simulink model "RobotX_ss_acousticsSingle_DockT_1024"  (R2014a)
settings: Solver=FixedStepDiscrete  StartTime=0.0  StopTime=inf  FixedStep=.25  RelTol=1e-3
undefined symbols (not defined in the file): Com1, Com2, Com3, Com4, DiscIntNeverNeededParam, standard
libraries: xpcseriallib x42, slrtlib x7, simulink x6, speedgoatlib x2, dspmtrx3 x1, speedgoatlib_IO102 x1
(part 3 of 4)

== system RobotX_ss_acousticsSingle_DockT_1024/Sensors/1024 Comms/Pi Nav Send ==
  Parameters : Inport
  ASCII Encode 3 : xpcseriallib/ASCII Encode   format="{\"Valid\":%d, \"Mode\":%d, \"Length\":%d, \"Activate\":%d, \"Waypoints\":[%f, %f, %f, %f, %f, %f, %f, %f, %f, %f, %f, %f, %f, %f, %f, %f, %f, %f, %f, %f, %f, %f, %f, %f]} \\r\\n"  nvars=28  maxlength=1000  vartypes={ 'double' }
  Bus Selector : BusSelector  OutputSignals=Outputs.Navigation Outputs.Valid,Outputs.Navigation Outputs.Control Mode,Outputs.Navigation Outputs.Data,Outputs.Acoustic Active
  Data Update1 : MATLAB Function  Commented=on  TreatAsAtomicUnit=on
  Data Update2 : MATLAB Function  TreatAsAtomicUnit=on
  LCM Complete Encode : xpcseriallib/ASCII Encode   Commented=on  format="{\"Valid\":%d, \"Mode\":%d, \"Length\":%d, \"Activate\":%d, \"Waypoints\":[%f, %f, %f, %f, %f, %f, %f, %f, %f, %f, %f, %f, %f, %f, %f, %f, %f, %f, %f, %f, %f, %f, %f, %f]} \\r\\n"  nvars=28  maxlength=1000  vartypes={ 'double' }
  Serial Send : Outport
  wires:
  Parameters/1 -> Bus Selector/1
  ASCII Encode 3/1 -> Serial Send/1
  Bus Selector/1 -> Data Update2/1(Valid)  "<Valid>"
  Bus Selector/2 -> Data Update2/2(ControlMode)  "<Control Mode>"
  Bus Selector/3 -> Data Update2/3(Data)  "<Data>"
  Data Update2/21(D17) -> ASCII Encode 3/21
  Data Update2/20(D16) -> ASCII Encode 3/20
  Data Update2/19(D15) -> ASCII Encode 3/19
  Data Update2/4(A) -> ASCII Encode 3/4
  Data Update2/2(C) -> ASCII Encode 3/2
  Data Update2/18(D14) -> ASCII Encode 3/18
  Data Update2/16(D12) -> ASCII Encode 3/16
  Data Update2/7(D3) -> ASCII Encode 3/7
  Data Update2/6(D2) -> ASCII Encode 3/6
  Data Update2/5(D1) -> ASCII Encode 3/5
  Data Update2/17(D13) -> ASCII Encode 3/17
  Data Update2/9(D5) -> ASCII Encode 3/9
  Data Update2/10(D6) -> ASCII Encode 3/10
  Data Update2/24(D20) -> ASCII Encode 3/24
  Data Update2/23(D19) -> ASCII Encode 3/23
  Data Update2/28(D24) -> ASCII Encode 3/28
  Data Update2/26(D22) -> ASCII Encode 3/26
  Data Update2/25(D21) -> ASCII Encode 3/25
  Data Update2/3(L) -> ASCII Encode 3/3
  Data Update2/27(D23) -> ASCII Encode 3/27
  Data Update2/8(D4) -> ASCII Encode 3/8
  Data Update2/11(D7) -> ASCII Encode 3/11
  Data Update2/13(D9) -> ASCII Encode 3/13
  Data Update2/12(D8) -> ASCII Encode 3/12
  Data Update2/14(D10) -> ASCII Encode 3/14
  Data Update2/22(D18) -> ASCII Encode 3/22
  Data Update2/15(D11) -> ASCII Encode 3/15
  Bus Selector/4 -> Data Update2/4(Activate)  "<Acoustic Active>"
  Data Update2/1(V) -> ASCII Encode 3/1
  Data Update1/1(V) -> LCM Complete Encode/1
  Data Update1/2(C) -> LCM Complete Encode/2
  Data Update1/6(D2) -> LCM Complete Encode/6
  Data Update1/7(D3) -> LCM Complete Encode/7
  Data Update1/8(D4) -> LCM Complete Encode/8
  Data Update1/5(D1) -> LCM Complete Encode/5
  Data Update1/9(D5) -> LCM Complete Encode/9
  Data Update1/10(D6) -> LCM Complete Encode/10
  Data Update1/11(D7) -> LCM Complete Encode/11
  Data Update1/12(D8) -> LCM Complete Encode/12
  Data Update1/13(D9) -> LCM Complete Encode/13
  Data Update1/18(D14) -> LCM Complete Encode/18
  Data Update1/15(D11) -> LCM Complete Encode/15
  Data Update1/20(D16) -> LCM Complete Encode/20
  Data Update1/21(D17) -> LCM Complete Encode/21
  Data Update1/19(D15) -> LCM Complete Encode/19
  Data Update1/14(D10) -> LCM Complete Encode/14
  Data Update1/16(D12) -> LCM Complete Encode/16
  Data Update1/22(D18) -> LCM Complete Encode/22
  Data Update1/23(D19) -> LCM Complete Encode/23
  Data Update1/24(D20) -> LCM Complete Encode/24
  Data Update1/25(D21) -> LCM Complete Encode/25
  Data Update1/27(D23) -> LCM Complete Encode/27
  Data Update1/26(D22) -> LCM Complete Encode/26
  Data Update1/28(D24) -> LCM Complete Encode/28
  Data Update1/3(L) -> LCM Complete Encode/3
  Data Update1/4(A) -> LCM Complete Encode/4
  Data Update1/17(D13) -> LCM Complete Encode/17

== system RobotX_ss_acousticsSingle_DockT_1024/Sensors/1024 Comms/Subsystem ==
  Bus Creator : BusCreator  Inputs=3
  Bus Creator1 : BusCreator  Inputs=2
  Bus Creator2 : BusCreator  Inputs=2
  Constant : Constant  Value=zeros(12,1)
  Constant1 : Constant  Value=zeros(12,1)
  Constant2 : Constant  Value=zeros(4,1)
  Constant3 : Constant  Value=zeros(4,1)
  Constant4 : Constant  Value=zeros(4,1)
  Fake Panda : Outport
  wires:
  Constant/1 -> Bus Creator1/1  "Distances"
  Constant1/1 -> Bus Creator1/2  "Angles"
  Constant2/1 -> Bus Creator/1  "Color"
  Constant3/1 -> Bus Creator/2  "Probability"
  Constant4/1 -> Bus Creator/3  "idx"
  Bus Creator1/1 -> Bus Creator2/1  "Landmarks"
  Bus Creator/1 -> Bus Creator2/2  "Color data"
  Bus Creator2/1 -> Fake Panda/1  "Lidar Data Input"

== system RobotX_ss_acousticsSingle_DockT_1024/Sensors/1024 Comms/UTC Timer ==
  Start Time : Inport
  MATLAB Function : MATLAB Function  TreatAsAtomicUnit=on
  Real Time : Outport
  wires:
  Start Time/1 -> MATLAB Function/1(inTime)
  MATLAB Function/1(timeOut) -> Real Time/1

== system RobotX_ss_acousticsSingle_DockT_1024/Sensors/1024 Comms/data log ==
  Sensors signal : Inport
  Bus to Vector : BusToVector
  Read : DataStoreRead  DataStoreName=PingPose
  Scope 2 : slrtlib/Displays and Logging/Scope   scopeno=2  scopetype=File  autostart=on  viewmode=Graphical redraw  formatstr='%15.6f'  grid=on  ylimits=[0,0]  nosamples=250  noprepostsamples=0  interleave=1  triggermode=FreeRun  triggersignal=1  trigsignalfromport=off  triggerlevel=0.0  triggerslope=Either  triggerscope=1  triggersample=0  filename=NAL1_<%%%>1.dat  mode=Commit  writesize=512  autorestart=on  dynamicfilemode=on  maxwritefilesize=512*1024^2
  Scope 4 : slrtlib/Displays and Logging/Scope   scopeno=1  scopetype=File  autostart=on  viewmode=Graphical redraw  formatstr='%15.6f'  grid=on  ylimits=[0,0]  nosamples=250  noprepostsamples=0  interleave=1  triggermode=FreeRun  triggersignal=1  trigsignalfromport=off  triggerlevel=0.0  triggerslope=Either  triggerscope=1  triggersample=0  filename=pPos_<%%%>1.dat  mode=Commit  writesize=512  autorestart=on  dynamicfilemode=on  maxwritefilesize=512*1024^2
  wires:
  Sensors signal/1 -> Bus to Vector/1
  Bus to Vector/1 -> Scope 2/1
  Read/1 -> Scope 4/1

== system RobotX_ss_acousticsSingle_DockT_1024/Main FSM/Acoustic Single Point FSM/Acoustics Orient/Output Heirarchy ==
  Data : Inport
  Sensors : Inport  Port=2
  Acoustic Active : Constant
  Bus Creator2 : BusCreator  Inputs=3
  Bus Creator3 : BusCreator  Inputs=3
  Bus Creator5 : BusCreator  Inputs=2
  Constant : Constant
  Constant3 : Constant
  Lidar Mode : Constant
  Outputs : Outport
  wires:
  Sensors/1 -> Bus Creator5/2  "Sensors"
  Bus Creator5/1 -> Outputs/1  "Output Signals"
  Constant/1 -> Bus Creator2/1  "Valid"
  Constant3/1 -> Bus Creator2/2  "Control Mode"
  Data/1 -> Bus Creator2/3  "Data"
  Bus Creator2/1 -> Bus Creator3/1  "Navigation Outputs"
  Acoustic Active/1 -> Bus Creator3/2  "Acoustic Active"
  Lidar Mode/1 -> Bus Creator3/3  "Lidar Mode"
  Bus Creator3/1 -> Bus Creator5/1  "Outputs"

== system RobotX_ss_acousticsSingle_DockT_1024/Main FSM/Acoustic Single Point FSM/Move/Output Reassign ==
  Vaild : Inport
  Data : Inport  Port=2
  Sensors : Inport  Port=3
  Acoustic Active : Constant  Value=0
  Bus Creator2 : BusCreator  Inputs=3
  Bus Creator3 : BusCreator  Inputs=3
  Bus Creator5 : BusCreator  Inputs=2
  Constant3 : Constant  Value=0
  Lidar Mode : Constant  Value=0
  Outputs : Outport
  wires:
  Sensors/1 -> Bus Creator5/2  "Sensors"
  Bus Creator5/1 -> Outputs/1  "Output Signals"
  Vaild/1 -> Bus Creator2/1  "Valid"
  Constant3/1 -> Bus Creator2/2  "Control Mode"
  Data/1 -> Bus Creator2/3  "Data"
  Bus Creator2/1 -> Bus Creator3/1  "Navigation Outputs"
  Acoustic Active/1 -> Bus Creator3/2  "Acoustic Active"
  Lidar Mode/1 -> Bus Creator3/3  "Lidar Mode"
  Bus Creator3/1 -> Bus Creator5/1  "Outputs"

== system RobotX_ss_acousticsSingle_DockT_1024/Main FSM/Acoustic Single Point FSM/Report/Output Heirarchy ==
  Sensors : Inport
  Data : Inport  Port=2
  Acoustic Active : Constant
  Bus Creator2 : BusCreator  Inputs=3
  Bus Creator3 : BusCreator  Inputs=3
  Bus Creator5 : BusCreator  Inputs=2
  Constant : Constant
  Constant3 : Constant
  Lidar Mode : Constant
  Outputs : Outport
  wires:
  Sensors/1 -> Bus Creator5/2  "Sensors"
  Bus Creator5/1 -> Outputs/1  "Output Signals"
  Constant/1 -> Bus Creator2/1  "Valid"
  Constant3/1 -> Bus Creator2/2  "Control Mode"
  Data/1 -> Bus Creator2/3  "Data"
  Bus Creator2/1 -> Bus Creator3/1  "Navigation Outputs"
  Acoustic Active/1 -> Bus Creator3/2  "Acoustic Active"
  Lidar Mode/1 -> Bus Creator3/3  "Lidar Mode"
  Bus Creator3/1 -> Bus Creator5/1  "Outputs"

== system RobotX_ss_acousticsSingle_DockT_1024/Main FSM/Docking/Docking/Output Heirarchy ==
  Data : Inport
  Sensors : Inport  Port=2
  Acoustic Active : Constant  Value=0
  Bus Creator2 : BusCreator  Inputs=3
  Bus Creator3 : BusCreator  Inputs=3
  Bus Creator5 : BusCreator  Inputs=2
  Constant : Constant
  Constant3 : Constant
  Lidar Mode : Constant  Value=2
  Outputs : Outport
  wires:
  Sensors/1 -> Bus Creator5/2  "Sensors"
  Bus Creator5/1 -> Outputs/1  "Output Signals"
  Constant/1 -> Bus Creator2/1  "Valid"
  Constant3/1 -> Bus Creator2/2  "Control Mode"
  Data/1 -> Bus Creator2/3  "Data"
  Bus Creator2/1 -> Bus Creator3/1  "Navigation Outputs"
  Acoustic Active/1 -> Bus Creator3/2  "Acoustic Active"
  Lidar Mode/1 -> Bus Creator3/3  "Lidar Mode"
  Bus Creator3/1 -> Bus Creator5/1  "Outputs"

== system RobotX_ss_acousticsSingle_DockT_1024/Main FSM/Docking/GPS Move/Output Reassign ==
  Vaild : Inport
  Data : Inport  Port=2
  Sensors : Inport  Port=3
  Acoustic Active : Constant  Value=0
  Bus Creator2 : BusCreator  Inputs=3
  Bus Creator3 : BusCreator  Inputs=3
  Bus Creator5 : BusCreator  Inputs=2
  Constant3 : Constant  Value=0
  Lidar Mode : Constant  Value=0
  Outputs : Outport
  wires:
  Sensors/1 -> Bus Creator5/2  "Sensors"
  Bus Creator5/1 -> Outputs/1  "Output Signals"
  Vaild/1 -> Bus Creator2/1  "Valid"
  Constant3/1 -> Bus Creator2/2  "Control Mode"
  Data/1 -> Bus Creator2/3  "Data"
  Bus Creator2/1 -> Bus Creator3/1  "Navigation Outputs"
  Acoustic Active/1 -> Bus Creator3/2  "Acoustic Active"
  Lidar Mode/1 -> Bus Creator3/3  "Lidar Mode"
  Bus Creator3/1 -> Bus Creator5/1  "Outputs"

== system RobotX_ss_acousticsSingle_DockT_1024/Main FSM/Docking/Reverse/Output Heirarchy ==
  Sensors : Inport
  Acoustic Active : Constant  Value=0
  Bus Creator2 : BusCreator  Inputs=3
  Bus Creator3 : BusCreator  Inputs=3
  Bus Creator5 : BusCreator  Inputs=2
  Constant2 : Constant  Value=[-100; -100; zeros(22,1)]
  Constant3 : Constant
  Constant4 : Constant  Value=2
  Lidar Mode : Constant  Value=2
  Outputs : Outport
  wires:
  Sensors/1 -> Bus Creator5/2  "Sensors"
  Bus Creator5/1 -> Outputs/1  "Output Signals"
  Constant3/1 -> Bus Creator2/1  "Valid"
  Constant4/1 -> Bus Creator2/2  "Control Mode"
  Constant2/1 -> Bus Creator2/3  "Data"
  Bus Creator2/1 -> Bus Creator3/1  "Navigation Outputs"
  Acoustic Active/1 -> Bus Creator3/2  "Acoustic Active"
  Lidar Mode/1 -> Bus Creator3/3  "Lidar Mode"
  Bus Creator3/1 -> Bus Creator5/1  "Outputs"

== matlab function RobotX_ss_acousticsSingle_DockT_1024/Main FSM/Docking/Docking/MATLAB Function ==
  data: QuayHeading input; TargetPoints input; Finished output; X input; Data output; Y input; Psi input; Dist input; Angles input; Prob input; Time input; dockNum input
function [Finished,Data] = Orient(QuayHeading,TargetPoints,X,Y,Psi,Dist,Angles,Prob,Time,dockNum)
%Written by Dylan DeGaetano on September 2, 2014
%Last Edited By Anderson Lebbad on September 19 2014

%This function passes the current pose data with the requrested heading
%so that the boat is facing the Quay wall.This task must be in station
%keeping mode
%
%Anderson's edit moved the orient within this function and adjusts the code
%to work better with sensing information

% 10/21 Edit: Correlates the estimated NED coord of the found symbol with
% known locations found through Ivan's map and proceeds to those locations

% Input TargetPoint is a 10x2 matrix of NED coords structured as follows
% [Observation Point; Dock1Start; Dock1Inter; Dock1Fin; Dock2Start;
% Dock2Inter; Dock2Fin; Dock3Start; Dock3Inter; Dock3Fin] where the bay
% numbers go from left to right

%work aound for communication issue
idx = Prob(4);
% Holdpose = station keeping point that we want to get to
% Pose = which waypoint to head to
% posIdx = which docking symbol position it is @
% 1 = Left, 2 = Middle, 3 = Right
% recognized = flag for if position of dock is found

persistent holdPose pos posIdx recognized

% If not to hold position
if isempty(holdPose)
    holdPose = [TargetPoints(1,:) QuayHeading]; % Initialize with Observation Points
    pos = 0;
    posIdx = 0;
    recognized = 0;
end

DistM=Dist(1)/100; % CM to M
Finished = 0; % Task not completed

%Initialize Data variable
Data = zeros(24,1); % 24x1 Array of Zeros


if idx(1) ~= 0 && recognized == 0
    %Calculate the NED coordinate of the found symbol
    TargetX = X+DistM(idx(1))*cos((Psi+Angles(idx(1)))*pi/180);
    TargetY = Y+DistM(idx(1))*sin((Psi+Angles(idx(1)))*pi/180);
    
    % Since the quay wall is very well aligned with EW directions,
    % correlate the estimated E coord of the found symbol with one of
    % the known bay positions
    bayEPos = [TargetPoints(4,2); TargetPoints(7,2); TargetPoints(10,2)];
    PosDiff = bayEPos - TargetY;
    [~,posIdx] = min(PosDiff);
    
    % Flag symbol as recognized
    recognized = 1; % Ensure that this calculation is not made again after the dock symbol pos is found/calculated
    
    % Begin proceeding to first position
    pos = 1;
end

if pos == 1
        %Set destination in front of dock to line up
        holdPose(1) = TargetPoints(pos+posIdx+2^(posIdx-1),1); % North
        holdPose(2) = TargetPoints(pos+posIdx+2^(posIdx-1),2); % East
    
    l1norm = abs(X-holdPose(1))+abs(Y-holdPose(2)); % calculate range to point we want to get to
    
    if l1norm < 2 % 2 metters
        % If within range, then flag first position complete and begin
        % proceeding to the hext position
        pos = 2;
    end
elseif pos == 2
        % Set intermediate point between start and finish
        holdPose(1) = TargetPoints(pos+posIdx+2^(posIdx-1),1); % North
        holdPose(2) = TargetPoints(pos+posIdx+2^(posIdx-1),2); % East
    
    l2norm = abs(X-holdPose(1)) + abs(Y-holdPose(2));
    
    if l2norm < 2
        % If within range, then flag second position complete and begin
        % proceeding to the hext position
        pos = 3;
    end
elseif pos == 3
        % Set final docking point
        holdPose(1) = TargetPoints(pos+posIdx+2^(posIdx-1),1); % North
        holdPose(2) = TargetPoints(pos+posIdx+2^(posIdx-1),2); % East
    
    l3norm = abs(X-holdPose(1)) + abs(Y-holdPose(2));
    
    if l3norm < 2
        holdPose = [X Y QuayHeading];
        Finished = 1;
    end
end

if Time >= 120 && recognized == 0
    % If symbol cannot be found within 60 seconds, proceed to middle bay
    posIdx = dockNum;
    recognized = 1;
end

holdPose(3) = QuayHeading;

Data(1) = holdPose(1);
Data(2) = holdPose(2);
Data(3) = holdPose(3);

== matlab function RobotX_ss_acousticsSingle_DockT_1024/Sensors/1020 Comms/MATLAB Function1 ==
  data: Valid input; Time input; asciiSEA output; Lat input; Long input; Color input; Depth input
% This function creates the underwater search message to be sent from 
% Speedgoat in ascii code
% Written by: Edward Zhu
% Date: 9/17/14

function asciiSEA = asciiSEAEncoder(Valid, Time, Lat, Long, Color, Depth)

% Initialize output message vector as the serial output block expects 128
% character message
asciiSEA = uint8(zeros(1,128));

% Convert static strings to ascii code
asciiMsgID = uint8('$RXSEA,');
asciiComma = uint8(',');
asciiDeciPt = uint8('.');
if Valid == 1
    if Lat >= 0
        asciiNS = uint8('N,');
    else
        Lat = -Lat;
        asciiNS = uint8('S,');
    end
    if Long >= 0
        asciiEW = uint8('E,');
    else
        Long = -Long;
        asciiEW = uint8('W,');
    end
else
    asciiNS = [32 asciiComma];
    asciiEW = [32 asciiComma];
end
asciiTeamID = uint8('FAUVU,');
asciiMsgEnd = uint8('*');
asciiMsgCRLF = [13 10];

% Convert UTC Time input (hhmmss) into ascii code
asciiTime = uint8(zeros(1,7));
asciiTime(7) = asciiComma;

for timeChar = 1:6
    asciiTime(timeChar) = floor(mod(Time,10^(7-timeChar))/...
        10^(6-timeChar)) + 48;
end

% Convert buoy color to ascii code (1 = R, 2 = G, 3 = B, 4 = W, 5 = K)
asciiColor = [uint8(32) asciiComma]; % Initialize as whitespace in case no buoy is found
if Valid == 1
    if Color == 1
        asciiColor(1) = uint8('R');
    elseif Color == 2
        asciiColor(1) = uint8('G');
    elseif Color == 3
        asciiColor(1) = uint8('B');
    elseif Color == 4
        asciiColor(1) = uint8('W');
    elseif Color == 5
        asciiColor(1) = uint8('K');
    end
end
% Convert latitude (dd.mmmmmm) into ascii code
asciiLat = uint8(zeros(1,10)+32); % Initialize as whitespace in case no buoy is found
asciiLat(10) = asciiComma;

% Only output values if valid bit is high
if Valid == 1
    asciiLat(3) = asciiDeciPt;
    latInt = floor(Lat);
    for latIntChar = 1:2
        asciiLat(latIntChar) = floor(mod(latInt,10^(3-latIntChar))/...
            10^(2-latIntChar)) + 48;
    end
    
    latDeci = mod(Lat,latInt) * 10^6;
    for latDeciChar = 1:6
        asciiLat(latDeciChar+3) = floor(mod(latDeci,10^(7-latDeciChar))/...
            10^(6-latDeciChar)) + 48;
    end
end

% Convert longitude (ddd.mmmmmm) into ascii code
asciiLong = uint8(zeros(1,11)+32); % Initialize as whitespace in case no buoy is found
asciiLong(11) = asciiComma;

% Only output values if valid bit is high
if Valid == 1
    asciiLong(4) = asciiDeciPt;
    longInt = floor(Long);
    for longIntChar = 1:3
        asciiLong(longIntChar) = floor(mod(longInt,10^(4-longIntChar))/...
            10^(3-longIntChar)) + 48;
    end
    
    longDeci = mod(Long,longInt) * 10^6;
    for longDeciChar = 1:6
        asciiLong(longDeciChar+4) = floor(mod(longDeci,10^(7-longDeciChar))/...
            10^(6-longDeciChar)) + 48;
    end
end

% Convert depth (m) (##.##) into ascii
asciiDepth = uint8(zeros(1,6)+32); % Initialize as whitespace in case no buoy is found
asciiDepth(6) = asciiMsgEnd;

% Only output values if valid bit is high
if Valid == 1
    asciiDepth(3) = asciiDeciPt;
    depthInt = floor(Depth);
    for depthIntChar = 1:2
        asciiDepth(depthIntChar) = floor(mod(depthInt,10^(3-depthIntChar))/...
            10^(2-depthIntChar)) + 48;
    end
    
    depthDeci = mod(Depth,depthInt) * 10^2;
    for depthDeciChar = 1:2
        asciiDepth(depthDeciChar+3) = floor(mod(depthDeci,10^(3-depthDeciChar))/...
            10^(2-depthDeciChar)) + 48;
    end
end

% Concat individual ascii arrays into one array
asciiPreChkSum = cat(2,asciiMsgID,asciiTime,asciiTeamID,asciiColor,...
    asciiLat,asciiNS,asciiLong,asciiEW,asciiDepth);

% Calculate the checksum of the message from the '$' to the '*' and convert
% to hex
chkSum = uint8(0);

for chksumChar = 1:(length(asciiPreChkSum)-2)
    chkSum = bitxor(chkSum,asciiPreChkSum(chksumChar+1));
end

% Convert the checksum to ascii
chkSum = dec2hex(chkSum);
asciiChkSum = uint8(zeros(1,length(chkSum))+32);
for i = 1:length(chkSum)
    asciiChkSum(i) = uint8(chkSum(i));
end

% Concat the checksum and the '/r/n' to the end of the message
asciiPostChkSum = cat(2,asciiPreChkSum,asciiChkSum,asciiMsgCRLF);

% Output the final message
asciiSEA(1:length(asciiPostChkSum)) = asciiPostChkSum;

== system RobotX_ss_acousticsSingle_DockT_1024/Main FSM/Start//Speedgate/Aim/Output Heirarchy ==
  Data : Inport
  Sensors : Inport  Port=2
  Acoustic Active : Constant  Value=0
  Bus Creator2 : BusCreator  Inputs=3
  Bus Creator3 : BusCreator  Inputs=3
  Bus Creator5 : BusCreator  Inputs=2
  Constant : Constant
  Constant3 : Constant
  Lidar Mode : Constant
  Outputs : Outport
  wires:
  Sensors/1 -> Bus Creator5/2  "Sensors"
  Bus Creator5/1 -> Outputs/1  "Output Signals"
  Constant/1 -> Bus Creator2/1  "Valid"
  Constant3/1 -> Bus Creator2/2  "Control Mode"
  Data/1 -> Bus Creator2/3  "Data"
  Bus Creator2/1 -> Bus Creator3/1  "Navigation Outputs"
  Acoustic Active/1 -> Bus Creator3/2  "Acoustic Active"
  Lidar Mode/1 -> Bus Creator3/3  "Lidar Mode"
  Bus Creator3/1 -> Bus Creator5/1  "Outputs"

== system RobotX_ss_acousticsSingle_DockT_1024/Main FSM/Start//Speedgate/Dead Reckon/Output Reassign ==
  Vaild : Inport
  Data : Inport  Port=2
  Sensors : Inport  Port=3
  Acoustic Active : Constant  Value=0
  Bus Creator2 : BusCreator  Inputs=3
  Bus Creator3 : BusCreator  Inputs=3
  Bus Creator5 : BusCreator  Inputs=2
  Constant3 : Constant  Value=0
  Lidar Mode : Constant  Value=3
  Outputs : Outport
  wires:
  Sensors/1 -> Bus Creator5/2  "Sensors"
  Bus Creator5/1 -> Outputs/1  "Output Signals"
  Vaild/1 -> Bus Creator2/1  "Valid"
  Constant3/1 -> Bus Creator2/2  "Control Mode"
  Data/1 -> Bus Creator2/3  "Data"
  Bus Creator2/1 -> Bus Creator3/1  "Navigation Outputs"
  Acoustic Active/1 -> Bus Creator3/2  "Acoustic Active"
  Lidar Mode/1 -> Bus Creator3/3  "Lidar Mode"
  Bus Creator3/1 -> Bus Creator5/1  "Outputs"

== system RobotX_ss_acousticsSingle_DockT_1024/Main FSM/Start//Speedgate/GPS Move/Output Reassign ==
  Vaild : Inport
  Data : Inport  Port=2
  Sensors : Inport  Port=3
  Acoustic Active : Constant  Value=0
  Bus Creator2 : BusCreator  Inputs=3
  Bus Creator3 : BusCreator  Inputs=3
  Bus Creator5 : BusCreator  Inputs=2
  Constant3 : Constant  Value=0
  Lidar Mode : Constant  Value=0
  Outputs : Outport
  wires:
  Sensors/1 -> Bus Creator5/2  "Sensors"
  Bus Creator5/1 -> Outputs/1  "Output Signals"
  Vaild/1 -> Bus Creator2/1  "Valid"
  Constant3/1 -> Bus Creator2/2  "Control Mode"
  Data/1 -> Bus Creator2/3  "Data"
  Bus Creator2/1 -> Bus Creator3/1  "Navigation Outputs"
  Acoustic Active/1 -> Bus Creator3/2  "Acoustic Active"
  Lidar Mode/1 -> Bus Creator3/3  "Lidar Mode"
  Bus Creator3/1 -> Bus Creator5/1  "Outputs"

== system RobotX_ss_acousticsSingle_DockT_1024/Sensors/1024 Comms/Message Selector/HRT Message ==
  Parameters : Inport
  Time : Inport  Port=2
  Bus Selector : BusSelector  OutputSignals=Sensors.Navigation Message.GPS (LLA).Lat,Sensors.Navigation Message.GPS (LLA).Long,Sensors.Navigation Message.On/Off/RC/Auto,Main Task
  MATLAB Function : MATLAB Function  TreatAsAtomicUnit=on
  HRT Message : Outport
  wires:
  MATLAB Function/1(asciiHRT) -> HRT Message/1
  Parameters/1 -> Bus Selector/1
  Time/1 -> MATLAB Function/1(Time)
  Bus Selector/1 -> MATLAB Function/2(HRTLat)  "<Lat>"
  Bus Selector/2 -> MATLAB Function/3(HRTLong)  "<Long>"
  Bus Selector/3 -> MATLAB Function/4(HRTMode)  "<On/Off/RC/Auto>"
  Bus Selector/4 -> MATLAB Function/5(HRTTask)  "<Main Task>"

== system RobotX_ss_acousticsSingle_DockT_1024/Sensors/1024 Comms/Message Selector/HRTLIT Message ==
  Parameters : Inport
  Time : Inport  Port=2
  Bus Selector : BusSelector  OutputSignals=Sensors.Navigation Message.GPS (LLA).Lat,Sensors.Navigation Message.GPS (LLA).Long,Main Task,Sensors.Navigation Message.On/Off/RC/Auto
  Data Store Read1 : DataStoreRead  DataStoreName=ltSeq
  MATLAB Function : MATLAB Function  TreatAsAtomicUnit=on
  MATLAB Function1 : MATLAB Function  TreatAsAtomicUnit=on
  HRTLIT Message : Outport
  wires:
  MATLAB Function/1(asciiHRTLIT) -> HRTLIT Message/1
  Time/1 -> MATLAB Function/1(Time)
  Parameters/1 -> Bus Selector/1
  Bus Selector/3 -> MATLAB Function/4(HRTTask)  "<Main Task>"
  Bus Selector/2 -> MATLAB Function/3(HRTLong)  "<Long>"
  Bus Selector/1 -> MATLAB Function/2(HRTLat)  "<Lat>"
  Bus Selector/4 -> MATLAB Function/5(HRTMode)  "<On/Off/RC/Auto>"
  Data Store Read1/1 -> MATLAB Function1/1(ltSeq)
  MATLAB Function1/2(LITSequence) -> MATLAB Function/7(LITSequence)
  MATLAB Function1/1(LITValid) -> MATLAB Function/6(LITValid)

== system RobotX_ss_acousticsSingle_DockT_1024/Sensors/1024 Comms/Message Selector/HRTSEA Message ==
  Parameters : Inport
  Time : Inport  Port=2
  Bus Selector : BusSelector  OutputSignals=Sensors.Navigation Message.GPS (LLA).Lat,Sensors.Navigation Message.GPS (LLA).Long,Main Task,Sensors.Navigation Message.On/Off/RC/Auto
  Data Store Read3 : DataStoreRead  DataStoreName=pingerInfo
  MATLAB Function : MATLAB Function  TreatAsAtomicUnit=on
  MATLAB Function1 : MATLAB Function  TreatAsAtomicUnit=on
  HRTSEA Message : Outport
  wires:
  MATLAB Function/1(asciiHRTSEA) -> HRTSEA Message/1
  Parameters/1 -> Bus Selector/1
  Time/1 -> MATLAB Function/1(Time)
  Data Store Read3/1 -> MATLAB Function1/1(pingerInfo)
  Bus Selector/3 -> MATLAB Function/4(HRTTask)  "<Main Task>"
  Bus Selector/1 -> MATLAB Function/2(HRTLat)  "<Lat>"
  Bus Selector/2 -> MATLAB Function/3(HRTLong)  "<Long>"
  Bus Selector/4 -> MATLAB Function/5(HRTMode)  "<On/Off/RC/Auto>"
  MATLAB Function1/3(SEALong) -> MATLAB Function/8(SEALong)
  MATLAB Function1/2(SEALat) -> MATLAB Function/7(SEALat)
  MATLAB Function1/5(SEADepth) -> MATLAB Function/10(SEADepth)
  MATLAB Function1/4(SEAColor) -> MATLAB Function/9(SEAColor)
  MATLAB Function1/1(SEAValid) -> MATLAB Function/6(SEAValid)

== matlab function RobotX_ss_acousticsSingle_DockT_1024/Main FSM/Acoustic Single Point FSM/Report/writePingInfo ==
  data: acouX input; acouY input; Depth input; NED_Origin input; pingerInfo output; AcousticPose1 input; colorQuad input
function pingerInfo = writePingInfo(acouX,acouY,Depth,NED_Origin,AcousticPose1,colorQuad)
%Written By Anderson Lebbad on October 22, 2014
%Last Edited By:
%
%This function takes the info from the acoustic pose to create an estimate
%of pinger position in North East Down coordinates, then converts that to
%LLA. From here, a buoy color is chosen based off the quadrant, and the
%info is formatted for the message writing block - including the valid bit.

Psi = AcousticPose1(3);

%Quadrants -
%NE : 1
%SE : 2
%SW : 3
%NW : 4
Quad = round((mod(Psi,360)+45)/90);



%Color code-
%R : 1
%G : 2
%B : 3
%W : 4
%K : 5

switch Quad
    case 1
        color = colorQuad(1);
    case 2
        color = colorQuad(2);
    case 3
        color = colorQuad(3);
    otherwise
        color = colorQuad(4);
end

%Convert to LLA
LLA = ecef2lla(ned2ecef(NED_Origin'*pi/180,[acouX; acouY; 0]))*180/pi;

%Output
pingerInfo = [1, LLA(1), LLA(2), Depth, color];

end

function x_ecef = ned2ecef(ned_lla, x_ned)
% NED2ECEF 
% INPUT:
% 1) x_ned=[x,y,z]' (m) NED coordinates
% 2) ned_lla=[phi,lambda]' consiting of latitude phi (rad) and longitude lambda (rad) of NED origin
% OUTPUT:
% 1) x_ecef=[x,y,z]' (m) in earth-centered, earth-fixed coordinate system with the origin [phi,lambda]'

    phi = ned_lla(1);
    lambda = ned_lla(2);

    % transformation  matrix
    T = [-sin(phi)*cos(lambda) -sin(phi)*sin(lambda)  cos(phi)
         -sin(lambda)           cos(lambda)           0
          cos(phi)*cos(lambda)   cos(phi)*sin(lambda)  sin(phi)];
    
    x_ecef = T'*x_ned + lla2ecef([phi, lambda, 0]');
end

function [x_lla] = ecef2lla(x_ecef)
% ECEF2LLH Converts from earth-centered, earth-fixed Cartesian coordinates to latitude, longitude, and altitude
% INPUT: x_ecef=[x,y,z]' (m) earth-centered, earth-fixed Cartesian coordinates
% OUTPUT: x_lla=[phi, lambda, h]' (rad, rad, m) GPS coordinates
    a = 6378137; % equatorial radius of ellipsoid (semi-major axis) (m)
    b = 6356752; % polar axis radius of ellipsoid (semi-minor axis) (m)

    x = x_ecef(1);
    y = x_ecef(2);
    z = x_ecef(3);
    
    % define auxiliary parameters e and f
    f = (a-b)/a;
    e = f*(2-f);
    
    lambda = atan(y/x);
    phi = atan(inv(1-e^2)*z/sqrt(x^2+y^2));
    N = a/sqrt(1-(e*sin(phi))^2);
    h = sqrt(x^2+y^2)/cos(phi)-N;
    
    x_lla = [phi; lambda; h];
end

== matlab function RobotX_ss_acousticsSingle_DockT_1024/Main FSM/Acoustic Single Point FSM/Acoustics Orient/Ping Point ==
  data: acousticPose output; Deployed input; Finished output; X input; Y input; Psi input; HorizBearing input; ElapsedTime input; Data output
function [acousticPose,Finished,Data] = PingPoint(Deployed,X,Y,Psi,...
    HorizBearing,ElapsedTime)
%Written by Anderson Lebbad on September 12, 2014
%Last Edited: September 14 - waits for boom deployment

%This function causes the vessel to spin in place until a ping is detected,
%then orients itself towards the direction of the source of that ping

persistent holdPose Pinged aveHeading First aveXY

if isempty(holdPose)
    holdPose = [X Y Psi];
    Pinged = 0;
    aveHeading = [0 0];
    aveXY = [0 0];
    First = 1;
end

%Initialize Data variable
Data = zeros(24,1);
Finished = 0;

%Angular offset (indirect rate control)
offset = 5;

%Wait for the boom to be lowered
if Deployed == 1
    %If the boat has not heard a ping yet, spin
    if Pinged == 0
        holdPose(3) = mod(Psi + offset,360);
    end
    
    %If the ping is less than 250 milliseconds (a timestep) then point at the
    %direction of sound
    if ElapsedTime < 250 && abs(HorizBearing) < 35
        if (abs(HorizBearing) >= 15 || First)
            holdPose(3) = mod(Psi + HorizBearing,360);
            Pinged = 1;
            First = 0;
        end
        aveHeading(1) = (aveHeading(1)*aveHeading(2)+Psi+HorizBearing)/(aveHeading(2)+1);
        aveHeading(2) = aveHeading(2)+1;
        aveXY(1) = (aveXY(1)*(aveHeading(2)-1)+X)/aveHeading(2);
        aveXY(2) = (aveXY(2)*(aveHeading(2)-1)+Y)/aveHeading(2);
    end
end

acousticPose = [aveXY aveHeading(1)];

if aveHeading(2) >= 16
    Finished = 1;
end

%Set desired pose
Data(1) = holdPose(1);
Data(2) = holdPose(2);
Data(3) = holdPose(3);

== matlab function RobotX_ss_acousticsSingle_DockT_1024/Sensors/1024 Comms/Lidar Send/MATLAB Function ==
  data: symbol input; LidarMode output; MainMode input
function LidarMode = selectLidarMode(symbol,MainMode)
%Written By Anderson Lebbad on October 21, 2014
%Last Edited By:
%
%This function decides the lidar mode to select based on the current task
%and docking symbol of the day.

if MainMode == 4
    LidarMode = symbol+2;
else
    LidarMode = 7;
end

end

== matlab function RobotX_ss_acousticsSingle_DockT_1024/Course Selections/MATLAB Function1 ==
  data: bay1Offset input; bayNED output; bay2Offset input; bay3Offset input; obsX input; startX input; interX input; finX input; bay1Y input; bay2Y input; bay3Y input
function bayNED = fcn(bay1Offset,bay2Offset,bay3Offset,obsX,startX,interX,finX,bay1Y,bay2Y,bay3Y)

% Define the NED points for the docking bays as found from Ivan's map
% obsX = 76;
% startX = 78;
% interX = 82;
% finX = 86;
% bay1Y = -127.7;
% bay2Y = -121.8;
% bay3Y = -115.9;

% Add or subtract offsets based on actual execution of task
bayNED = [obsX bay2Y+bay2Offset;
   startX bay1Y+bay1Offset;
   interX bay1Y+bay1Offset;
   finX bay1Y+bay1Offset;
   startX bay2Y+bay2Offset;
   interX bay2Y+bay2Offset;
   finX bay2Y+bay2Offset;
   startX bay3Y+bay3Offset;
   interX bay3Y+bay3Offset;
   finX bay3Y+bay3Offset];

== matlab function RobotX_ss_acousticsSingle_DockT_1024/Sensors/1024 Comms/Message Selector/HRT Message/MATLAB Function ==
  data: Time input; asciiHRT output; HRTLat input; HRTLong input; HRTMode input; HRTTask input
% This function creates the heartbeat message to be sent from Speedgoat in
% ascii code
% Written by: Edward Zhu
% Date: 9/17/14

function asciiHRT = asciiHRTEncoder(Time, HRTLat, HRTLong, HRTMode, HRTTask)

% Initialize output message vector as the serial output block expects 128
% character message
asciiHRT = uint8(zeros(1,128));

% Convert static strings to ascii code
asciiHRTMsgID = uint8('$RXHRT,');
asciiComma = uint8(',');
asciiDeciPt = uint8('.');
if HRTLat >= 0
    asciiHRTNS = uint8('N,');
else
    HRTLat = -HRTLat;
    asciiHRTNS = uint8('S,');
end
if HRTLong >= 0
    asciiHRTEW = uint8('E,');
else
    HRTLong = -HRTLong;
    asciiHRTEW = uint8('W,');
end
asciiTeamID = uint8('FAUVU,');
asciiMsgEnd = uint8('*');
asciiMsgCRLF = [13 10];

% Convert UTC Time input (hhmmss) into ascii code
asciiTime = uint8(zeros(1,7));
asciiTime(7) = asciiComma;

for timeChar = 1:6
    asciiTime(timeChar) = floor(mod(Time,10^(7-timeChar))/...
        10^(6-timeChar)) + 48;
end

% Convert latitude (dd.mmmmmm) into ascii code
asciiHRTLat = uint8(zeros(1,10));
asciiHRTLat(10) = asciiComma;
asciiHRTLat(3) = asciiDeciPt;

HRTlatInt = floor(HRTLat);
for latIntChar = 1:2
    asciiHRTLat(latIntChar) = floor(mod(HRTlatInt,10^(3-latIntChar))/...
        10^(2-latIntChar)) + 48;
end

HRTlatDeci = mod(HRTLat,HRTlatInt) * 10^6;
for latDeciChar = 1:6
    asciiHRTLat(latDeciChar+3) = floor(mod(HRTlatDeci,10^(7-latDeciChar))/...
        10^(6-latDeciChar)) + 48;
end

% Convert longitude (ddd.mmmmmm) into ascii code
asciiHRTLong = uint8(zeros(1,11));
asciiHRTLong(11) = asciiComma;
asciiHRTLong(4) = asciiDeciPt;

HRTlongInt = floor(HRTLong);
for longIntChar = 1:3
    asciiHRTLong(longIntChar) = floor(mod(HRTlongInt,10^(4-longIntChar))/...
        10^(3-longIntChar)) + 48;
end

HRTlongDeci = mod(HRTLong,HRTlongInt) * 10^6;
for longDeciChar = 1:6
    asciiHRTLong(longDeciChar+4) = floor(mod(HRTlongDeci,10^(7-longDeciChar))/...
        10^(6-longDeciChar)) + 48;
end


% Convert vehicle mode into ascii (1 = RC, 2 = Auto)

% Auto On 
if HRTMode == 3 
    HRTOpMode = 2;
    asciiHRTMode = [uint8(HRTOpMode+48) asciiComma];
else
    HRTOpMode = 1;
    asciiHRTMode = [uint8(HRTOpMode+48) asciiComma];
end

% Convert vehicle task into ascii
HRTTask = HRTTask - 1; % FSM: Init = 1, SSGate = 2, SEA = 3, Dock = 4, LIT = 5, Obst = 6
if HRTTask ~= 1 || 2 || 3 || 4 || 5
    HRTOpTask = 1;
    asciiHRTTask = [uint8(HRTOpTask+48) asciiMsgEnd];
else
    asciiHRTTask = [uint8(HRTTask+48) asciiMsgEnd];
end

% Concat individual ascii arrays into one array
asciiHRTPreChkSum = cat(2,asciiHRTMsgID,asciiTime,asciiHRTLat,asciiHRTNS,asciiHRTLong,asciiHRTEW,...
    asciiTeamID,asciiHRTMode,asciiHRTTask);

% Calculate the checksum of the message from the '$' to the '*' and convert
% to hex
HRTchkSum = uint8(0);

for chksumChar = 1:(length(asciiHRTPreChkSum)-2)
    HRTchkSum = bitxor(HRTchkSum,asciiHRTPreChkSum(chksumChar+1));
end

% Convert the checksum to ascii
HRTchkSum = dec2hex(HRTchkSum);
asciiHRTChkSum = uint8(zeros(1,length(HRTchkSum))+32);
for i = 1:length(HRTchkSum)
    asciiHRTChkSum(i) = uint8(HRTchkSum(i));
end

% Concat the checksum and the '/r/n' to the end of the message
asciiHRTPostChkSum = cat(2,asciiHRTPreChkSum,asciiHRTChkSum,asciiMsgCRLF);

% Output the final message
asciiHRT(1:length(asciiHRTPostChkSum)) = asciiHRTPostChkSum;

== matlab function RobotX_ss_acousticsSingle_DockT_1024/Sensors/1024 Comms/Message Selector/HRTLIT Message/MATLAB Function ==
  data: Time input; HRTLat input; HRTLong input; HRTTask input; HRTMode input; LITValid input; asciiHRTLIT output; LITSequence input
function asciiHRTLIT = asciiHRTLITEncoder(Time,HRTLat,HRTLong,HRTTask,HRTMode,LITValid,LITSequence)
% Initialize output message vector as the serial output block expects 128
% character message
asciiHRTLIT = uint8(zeros(1,128));

asciiComma = uint8(',');
asciiDeciPt = uint8('.');
asciiTeamID = uint8('FAUVU,');
asciiMsgEnd = uint8('*');
asciiMsgCRLF = [13 10];

% Convert UTC Time input (hhmmss) into ascii code
asciiTime = uint8(zeros(1,7));
asciiTime(7) = asciiComma;

for timeChar = 1:6
    asciiTime(timeChar) = floor(mod(Time,10^(7-timeChar))/...
        10^(6-timeChar)) + 48;
end

%%%%%%%%%%%%%%%%%%%%%%%%%%%%%%%%%%%%%%%%%%%%%%%%%%%%%%%%%%%%%%%%%%%%
% Heartbeat message
% Convert static strings to ascii code
asciiHRTMsgID = uint8('$RXHRT,');
if HRTLat >= 0
    asciiHRTNS = uint8('N,');
else
    HRTLat = -HRTLat;
    asciiHRTNS = uint8('S,');
end
if HRTLong >= 0
    asciiHRTEW = uint8('E,');
else
    HRTLong = -HRTLong;
    asciiHRTEW = uint8('W,');
end

% Convert latitude (dd.mmmmmm) into ascii code
asciiHRTLat = uint8(zeros(1,10));
asciiHRTLat(10) = asciiComma;
asciiHRTLat(3) = asciiDeciPt;

HRTlatInt = floor(HRTLat);
for latIntChar = 1:2
    asciiHRTLat(latIntChar) = floor(mod(HRTlatInt,10^(3-latIntChar))/...
        10^(2-latIntChar)) + 48;
end

HRTlatDeci = mod(HRTLat,HRTlatInt) * 10^6;
for latDeciChar = 1:6
    asciiHRTLat(latDeciChar+3) = floor(mod(HRTlatDeci,10^(7-latDeciChar))/...
        10^(6-latDeciChar)) + 48;
end

% Convert longitude (ddd.mmmmmm) into ascii code
asciiHRTLong = uint8(zeros(1,11));
asciiHRTLong(11) = asciiComma;
asciiHRTLong(4) = asciiDeciPt;

HRTlongInt = floor(HRTLong);
for longIntChar = 1:3
    asciiHRTLong(longIntChar) = floor(mod(HRTlongInt,10^(4-longIntChar))/...
        10^(3-longIntChar)) + 48;
end

HRTlongDeci = mod(HRTLong,HRTlongInt) * 10^6;
for longDeciChar = 1:6
    asciiHRTLong(longDeciChar+4) = floor(mod(HRTlongDeci,10^(7-longDeciChar))/...
        10^(6-longDeciChar)) + 48;
end

% Convert vehicle mode into ascii (1 = RC, 2 = Auto)

% Auto On 
if HRTMode == 3 
    HRTOpMode = 2;
    asciiHRTMode = [uint8(HRTOpMode+48) asciiComma];
else
    HRTOpMode = 1;
    asciiHRTMode = [uint8(HRTOpMode+48) asciiComma];
end

% Convert vehicle task into ascii
HRTTask = HRTTask - 1; % FSM: Init = 1, SSGate = 2, SEA = 3, Dock = 4, LIT = 5, Obst = 6
if HRTTask ~= 1 || 2 || 3 || 4 || 5
    HRTOpTask = 1;
    asciiHRTTask = [uint8(HRTOpTask+48) asciiMsgEnd];
else
    asciiHRTTask = [uint8(HRTTask+48) asciiMsgEnd];
end

% Concat individual ascii arrays into one array
asciiHRTPreChkSum = cat(2,asciiHRTMsgID,asciiTime,asciiHRTLat,asciiHRTNS,asciiHRTLong,asciiHRTEW,...
    asciiTeamID,asciiHRTMode,asciiHRTTask);

% Calculate the checksum of the message from the '$' to the '*' and convert
% to hex
HRTchkSum = uint8(0);

for chksumChar = 1:(length(asciiHRTPreChkSum)-2)
    HRTchkSum = bitxor(HRTchkSum,asciiHRTPreChkSum(chksumChar+1));
end

% Convert the checksum to ascii
HRTchkSum = dec2hex(HRTchkSum);
asciiHRTChkSum = uint8(zeros(1,length(HRTchkSum))+32);
for i = 1:length(HRTchkSum)
    asciiHRTChkSum(i) = uint8(HRTchkSum(i));
end

% Concat the checksum and the '/r/n' to the end of the message
asciiHRTPostChkSum = cat(2,asciiHRTPreChkSum,asciiHRTChkSum,asciiMsgCRLF);

%%%%%%%%%%%%%%%%%%%%%%%%%%%%%%%%%%%%%%%%%%%%%%%%%%%%%%%%%%%%%%%%%%%%%

% Light tower message
asciiLITMsgID = uint8('$RXLIT,');

% Convert the light sequece into ascii code (1 = R, 2 = B, 3 = G)
asciiLITSeq = uint8(zeros(1,4)+32);
asciiLITSeq(4) = asciiMsgEnd;

if LITValid == 1
    for seqChar = 1:3
        if LITSequence(seqChar) == 1
            LITSequence(seqChar) = uint8('R');
        elseif LITSequence(seqChar) == 2
            LITSequence(seqChar) = uint8('B');
        elseif LITSequence(seqChar) == 3
            LITSequence(seqChar) = uint8('G');
        end
    end
    asciiLITSeq(1:3) = LITSequence;
end

% Concat individual ascii arrays into one array
asciiLITPreChkSum = cat(2,asciiLITMsgID,asciiTime,asciiTeamID,asciiLITSeq);

% Calculate the checksum of the message from the '$' to the '*' and convert
% to hex
LITchkSum = uint8(0);

for chksumChar = 1:(length(asciiLITPreChkSum)-2)
    LITchkSum = bitxor(LITchkSum,asciiLITPreChkSum(chksumChar+1));
end

% Convert the checksum to ascii
LITchkSum = dec2hex(LITchkSum);
asciiLITChkSum = uint8(zeros(1,length(LITchkSum))+32);
for i = 1:length(LITchkSum)
    asciiLITChkSum(i) = uint8(LITchkSum(i));
end

% Concat the checksum and the '/r/n' to the end of the message
asciiLITPostChkSum = cat(2,asciiLITPreChkSum,asciiLITChkSum,asciiMsgCRLF);

%%%%%%%%%%%%%%%%%%%%%%%%%%%%%%%%%%%%%%%%%%%%%%%%%%%%%%%%%%%%%%%%%%%%%%%%%%%

asciiHRTLITPostChkSum = cat(2,asciiHRTPostChkSum,asciiLITPostChkSum);
asciiHRTLIT(1:length(asciiHRTLITPostChkSum)) = asciiHRTLITPostChkSum;

== matlab function RobotX_ss_acousticsSingle_DockT_1024/Main FSM/Acoustic Single Point FSM/Report/MATLAB Function ==
  data: X input; Y input; Psi input; Data output
function Data  = Orient(X, Y, Psi)
%Written by Dylan DeGaetano on September 2, 2014
%Last Edited:Dylan DeGaetano on September 10,2014

%This function passes the current pose data added to the angle of the Light 
%buoy This stare forces the Boat to stare at the bouy.This task must be in station 
%keeping mode

persistent holdPose

if isempty(holdPose)
    holdPose = [X, Y, Psi];
end

%Initialize Data variable
Data = zeros(24,1);

%Set desired pose
Data(1) = holdPose(1);
Data(2) = holdPose(2);
Data(3) = holdPose(3);

end

== matlab function RobotX_ss_acousticsSingle_DockT_1024/Main FSM/Start//Speedgate/Aim/LLA to NED ==
  data: LLA input; GoalNED output; NED_origin input
function GoalNED = LLA2NEDfun(LLA,NED_origin)
%Written by Anderson Lebbad on September 20, 2014
%Last edited by:
%
%This function converts a target Latitude, Longitude, Altitude (LLA) point
%into North, East, Down (NED) coordinates

%First convert to earth centered, earth fixed frame
GoalECEF = lla2ecef([LLA*(pi/180), 0]');
%Then convert from ECEF to North East Down
GoalNEDvect = ecef2ned(NED_origin'*(pi/180),GoalECEF);
GoalNED = GoalNEDvect(1:2)';


end

function x_ecef = lla2ecef(x_lla)
% LLE2ECEF: Converts from geodetic latitude, longitude, and altitude to earth-centered earth-fixed Cartesian coordinates
% INPUT: latitude phi (rad), longitude lambda (rad), altitude h (m)
% OUTPUT: [x, y, z]' (m) earth-centered earth-fixed Cartesian coordinates
    a = 6378137; % equatorial radius of ellipsoid (semi-major axis) (m)
    b = 6356752; % polar axis radius of ellipsoid (semi-minor axis) (m)

    phi = x_lla(1);
    lambda = x_lla(2);
    h = x_lla(3);
    
    % auxiliar quantities f, e, and N
    f = (a-b)/a;
    e = f*(2-f);
    N = a/sqrt(1-(e*sin(phi))^2);
    x_ecef = [(N+h)*cos(phi)*cos(lambda); (N+h)*cos(phi)*sin(lambda); (N*(1-e^2)+h)*sin(phi)];
end

function [x_ned] = ecef2ned(ned_lla, x_ecef)
% ECEF2NED Converts from earth-centered, earth-fixed Cartesian coordinates to tangent plane
% INPUT:
% 1) x_ecef=[x,y,z]' (m) earth-centered, earth-fixed Cartesian coordinates
% 2) ned_lla=[phi,lambda]' consiting of latitude phi (rad), longitude lambda (rad) of NED origin
% OUTPUT:
% 1) x_ned=[x,y,z]' (m) in NED coordinate system with the origin [phi,lambda]'

    phi = ned_lla(1);
    lambda = ned_lla(2);

    % transformation  matrix
    T = [-sin(phi)*cos(lambda) -sin(phi)*sin(lambda)  cos(phi)
         -sin(lambda)           cos(lambda)           0
          cos(phi)*cos(lambda)   cos(phi)*sin(lambda)  sin(phi)];

     x_ned = T*(x_ecef-lla2ecef([phi, lambda, 0]')); % convert to NED
     x_ned(3) = -x_ned(3);
end

== matlab function RobotX_ss_acousticsSingle_DockT_1024/Main FSM/Start//Speedgate/Aim/MATLAB Function ==
  data: ssHeldHeading input; ssGateNED input; Data output
function Data  = Orient(ssHeldHeading,ssGateNED)
%Written by Dylan DeGaetano on September 2, 2014
%Last Edited:Dylan DeGaetano on September 10,2014

%This function passes the current pose data added to the angle of the Light 
%buoy This stare forces the Boat to stare at the bouy.This task must be in station 
%keeping mode

persistent holdPose

if isempty(holdPose)
    holdPose = [ssGateNED ssHeldHeading];
end

%Initialize Data variable
Data = zeros(24,1);

%Set desired pose
Data(1) = holdPose(1);
Data(2) = holdPose(2);
Data(3) = holdPose(3);

end

== matlab function RobotX_ss_acousticsSingle_DockT_1024/Main FSM/Start//Speedgate/Dead Reckon/Calculate Times ==
  data: pts input; u input; Data output
function Data = calcTimes(pts, u)
%Written by Anderson Lebbad on August 9, 2014
%Last Edited:

%Calculates times for the boat to get to points for a trajectory, and
%formats Data for communication

%Initialize
Data = zeros(24,1);
traj = zeros(8,3);

traj(:,1:2) = pts;

for k = 2:8
    %Calculate distance to travel from last point
    distTravel = sqrt(sum((pts(k-1,:)-pts(k,:)).^2));
    %Assume 1m per second speed
    traj(k,3) = traj(k-1,3) + distTravel;
    %Add time based off initial velocity to get to first point past initial
    if k == 2
        traj(k,3) = traj(k,3) + 2.5*abs(2-u);
    end
end


%Output Data
for i=1:8
    for j = 1:3
        Data(3*(i-1)+j) = traj(i,j);
    end
end

== matlab function RobotX_ss_acousticsSingle_DockT_1024/Main FSM/Start//Speedgate/Dead Reckon/Gate ==
  data: sglength input; ssHeldHeading input; Finished output; Valid output; X input; Y input; pts output
function [Finished, Valid, pts] = Gate(sglength,ssHeldHeading,X,Y)
%Written by Anderson Lebbad on August 9, 2014
%Last Edited by:

%This function sends a forward trajectory (from the initial heading read
%into it) until a landmark is found. Once the landmark is found, a
%trajectory is written to dodge around it.

pts = zeros(8,2);
Valid = 0;



persistent Found finPt
if isempty(Found)
    Found = 0;
    pts(1,1) = X + 5*cos(ssHeldHeading*pi/180);
    pts(1,2) = Y + 5*sin(ssHeldHeading*pi/180);
    pts(8,1) = X + sglength*cos(ssHeldHeading*pi/180);
    pts(8,2) = Y + sglength*sin(ssHeldHeading*pi/180);
    pts(2:7,:) = (1:6)'*(pts(8,:)-pts(1,:))/7+ones(6,1)*pts(1,:);
    Valid = 1;
    finPt = pts(8,:);
end

Finished = 0;

%Check to see how far the current pose is from the final point in the
%trajectory
range = abs(finPt(1)-X)+abs(finPt(2)-Y);


if range <= 10
    Finished = 1;
end

end

== matlab function RobotX_ss_acousticsSingle_DockT_1024/Main FSM/Main Enabler ==
  data: taskSelector output; initEn output; startgateEn output; acouEn output; dockEn output; termEn output; RCEn output; OnOffRCAuto input; initFin input; startgateFin input; acouFin input; dockFin input
function [taskSelector,initEn,startgateEn,acouEn,dockEn, termEn,RCEn] = taskEnabler(OnOffRCAuto,initFin,startgateFin,acouFin,dockFin)
%Written by Anderson Lebbad on September 13, 2014
%Last Edited by:

%Changes the value of MainMode and the enablers for the tasks within the
%Main FSM.

% Initialize enable signals
RCEn = 0;
initEn = 0;
startgateEn = 0;
termEn = 0;
acouEn = 0;
dockEn = 0;

% Set enable signals based on state completion
if initFin == 0
    initEn = 1;
    taskSelector = 1;
elseif OnOffRCAuto ~= 3
    RCEn = 1;
    taskSelector = 6;
elseif startgateFin == 0
    startgateEn = 1;
    taskSelector = 2;
elseif acouFin == 0
    acouEn = 1;
    taskSelector = 3;
elseif dockFin == 0
    dockEn = 1;
    taskSelector = 4;
else
    termEn = 1;
    taskSelector = 5;
end
